simulink model "planeModelFullModel"  (R2019b)
settings: Solver=VariableStepAuto  StartTime=0.0  StopTime=1000  RelTol=1e-3
values from neighbouring files (symbols this model uses):
  A = [   -0.322  0.052   0.028   -1.12   0.002 ... (first row only)    [Problem1.m]    (also in Task2.m)
  B = []    [Problem1.m]    (also in Task2.m = [0 0 0 0 7.5].')
  C = eye(2)    [Problem1.m]    (also in Task2.m = [eye(4), zeros(4,1)])
  D = []    [Problem1.m]    (also in Task2.m = [0 0 0 0].')
  g = 9.81    [Task2.m]
  k_dp = (2*zeta*wp - a_p1)/a_p2    [Task2.m]
  k_ic = 0.3*wc^2*V_g/g    [Task2.m]
  k_ip = -0.04    [Task2.m]
  k_pc = 2*zeta*wc*V_g/g    [Task2.m]
  k_pp = d_max/e_max*sign(a_p2)    [Task2.m]
  V_g = 580    [Task2.m]
libraries: simulink_extras x5, simulink x1
settings Model: Creator=sendt  LastModifiedBy=sendt

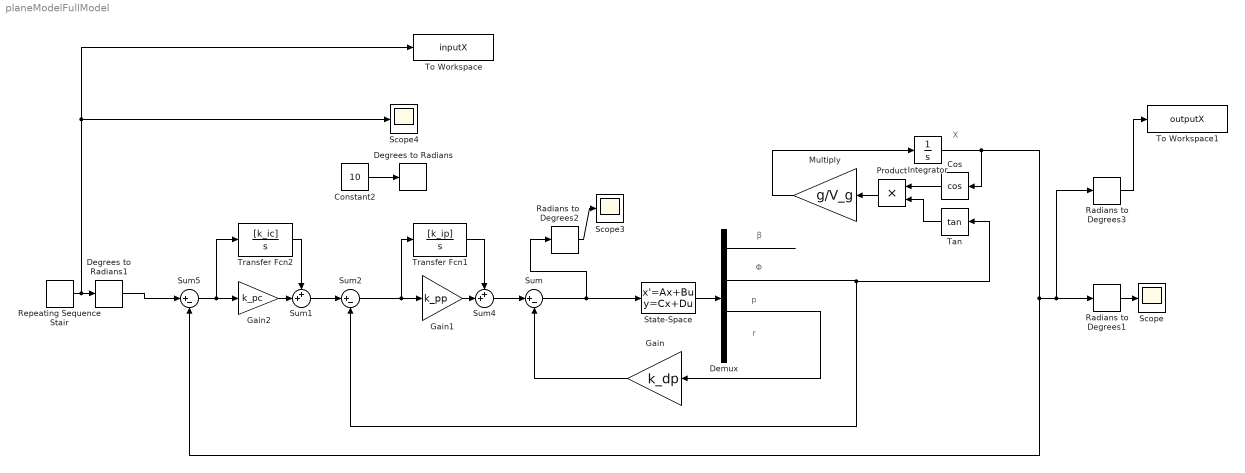
== system planeModelFullModel ==
  note: Χ
  note: r
  note: p
  note: Φ
  note: β
  Constant2 : Constant  Value=10
  Cos : Trigonometry  Operator=cos
  Degrees to Radians : simulink_extras/Transformations/Degrees to Radians
  Degrees to Radians1 : simulink_extras/Transformations/Degrees to Radians
  Demux : Demux
  Gain : Gain  Gain=k_dp
  Gain1 : Gain  Gain=k_pp
  Gain2 : Gain  Gain=k_pc
  Integrator : Integrator
  Multiply : Gain  Gain=g/V_g
  Product : Product
  Radians to Degrees1 : simulink_extras/Transformations/Radians to Degrees
  Radians to Degrees2 : simulink_extras/Transformations/Radians to Degrees
  Radians to Degrees3 : simulink_extras/Transformations/Radians to Degrees
  Repeating Sequence Stair : simulink/Sources/Repeating Sequence Stair  OutValues=[8 15 0 -3 0].'  tsamp=200  OutMin=[]  OutMax=[]  OutDataTypeStr=double  OutputDataTypeScalingMode=double  OutDataType=fixdt(0,8)  ConRadixGroup=Best Precision: Vector-wise  OutScaling=2^-12
  Scope : Scope
  Scope3 : Scope
  Scope4 : Scope
  State-Space : StateSpace  A=A  B=B  C=C  D=D  InitialCondition=0
  Sum : Sum  Inputs=|+-
  Sum1 : Sum  Inputs=++|
  Sum2 : Sum  Inputs=|+-
  Sum4 : Sum  Inputs=++|
  Sum5 : Sum  Inputs=|+-
  Tan : Trigonometry  Operator=tan
  To Workspace : ToWorkspace  VariableName=inputX  SaveFormat=Timeseries  SampleTime=-1
  To Workspace1 : ToWorkspace  VariableName=outputX  SaveFormat=Timeseries  SampleTime=-1
  Transfer Fcn1 : TransferFcn  Numerator=[k_ip]  Denominator=[1 0]
  Transfer Fcn2 : TransferFcn  Numerator=[k_ic]  Denominator=[1 0]
  wires:
  Gain/1 -> Sum/2
  Sum/1 -> Radians to Degrees2/1, State-Space/1
  Transfer Fcn2/1 -> Sum1/1
  Gain2/1 -> Sum1/2
  Sum5/1 -> Transfer Fcn2/1, Gain2/1
  Transfer Fcn1/1 -> Sum4/1
  Gain1/1 -> Sum4/2
  Repeating Sequence Stair/1 -> Scope4/1, To Workspace/1, Degrees to Radians1/1
  Integrator/1 -> Sum5/2, Radians to Degrees3/1, Radians to Degrees1/1, Cos/1
  Constant2/1 -> Degrees to Radians/1
  Sum4/1 -> Sum/1
  Sum2/1 -> Gain1/1, Transfer Fcn1/1
  Sum1/1 -> Sum2/1
  Degrees to Radians1/1 -> Sum5/1
  Radians to Degrees2/1 -> Scope3/1
  Radians to Degrees3/1 -> To Workspace1/1
  State-Space/1 -> Demux/1
  Demux/1 -> ?
  Demux/2 -> Tan/1, Sum2/2
  Demux/3 -> Gain/1
  Cos/1 -> Product/1
  Tan/1 -> Product/2
  Product/1 -> Multiply/1
  Multiply/1 -> Integrator/1
  Radians to Degrees1/1 -> Scope/1
